simulink model "lab4_S6_7_8_estimation_control"  (R2024b)
settings: Solver=ode23  StartTime=0.0  StopTime=sIn.simulation_time  RelTol=1e-3
values from neighbouring files (symbols this model uses):
  g = 9.81    [balrob_params.m]
  ms22g = 1/g    (= 0.101936799185)    [balrob_params.m]
  Ts = 1e-2    (= 0.01)    [balrob_params.m]
undefined symbols (not defined in the file or in its folder): DiscIntNeverNeededParam, Discrete, drv, feedback, filter, gbox, model, sens, sIn, Time, ua2tau, wheel
libraries: ctrlSharedLib x2
settings Model: Creator=Nihal  LastModifiedBy=Nihal

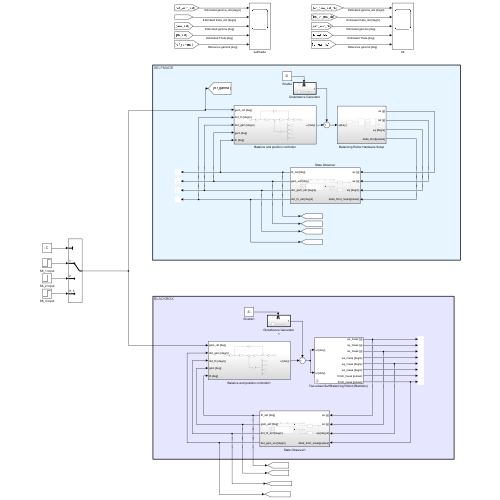
[thumbnail: Simulink's stored preview of the top-level diagram]
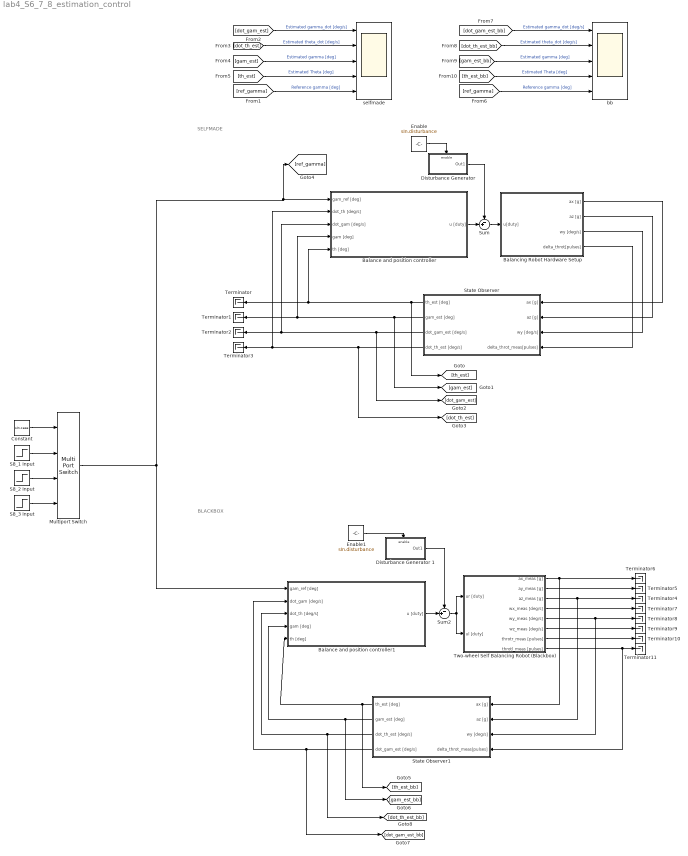
== system lab4_S6_7_8_estimation_control ==
  note: SELFMADE
  note: BLACKBOX
  Balance and position controller : Subsystem
  Balance and position controller1 : Subsystem
  Balancing Robot Hardware Setup : Subsystem
  Constant : Constant  Value=sIn.case
  "Disturbance Generator " : Subsystem  TreatAsAtomicUnit=on
  Disturbance Generator 1 : Subsystem  TreatAsAtomicUnit=on
  Enable : Constant  Value=sIn.disturbance
  Enable1 : Constant  Value=sIn.disturbance
  Multiport Switch : MultiPortSwitch  SaturateOnIntegerOverflow=off  InputSameDT=off
  S8_1 Input : Step  Time=0  After=0  SampleTime=0
  S8_2 Input : Step  Time=0  After=0.1/wheel.r  SampleTime=0
  S8_3 Input : Step  Time=0  After=0.1/wheel.r  SampleTime=0
  State Observer : Subsystem
  State Observer1 : Subsystem
  Sum : Sum  Inputs=-+|
  Sum2 : Sum  Inputs=-+|
  Terminator{,1..11} (12 alike) : Terminator
  "Two-wheel Self Balancing Robot (Blackbox) " : Subsystem  mask(Balancing robot (longitudinal + lateral dynamics)){initState=sIn.bb_ic, Ts=0.01}
      mask prompts: initState "Initial state [gam(0), psi(0), th(0), dot_gam(0), dot_psi(0), dot_th(0)]'"; Ts "Sample time:"
      mask help:
      | Balancing robot dynamic model.
      | Includes both the longitudinal and lateral (yaw) dynamics.
      mask init:
      | %% General parameters and conversion gains
      | 
      | %   gravity acc [m/s^2]
      | g = 9.81;
      | 
      | %   conversion gains
      | rpm2rads = 2*pi/60;         %   [rpm]   -> [rad/s]
      | rads2rpm = 60/2/pi;         %   [rad/s] -> [rpm]
      | rpm2degs = 360/60;          %   [rpm]   -> [deg/s]
      | degs2rpm = 60/360;          %   [deg/s] -> [rpm]
      | deg2rad = pi/180;           %   [deg]   -> [rad]
      | rad2deg = 180/pi;           %   [rad]   -> [deg]
      | g2ms2 = g;                  %   [acc_g] -> [m/s^2]
      | ms22g = 1/g;                %   [m/s^2] -> [acc_g]
      | ozin2Nm = 0.706e-2;         %   [oz*inch] -> [N*m]
      | 
      | 
      | %%  Battery data
      | 
      | %   electrical data
      | batt.UN = 11.1;     %   nominal voltage
      | 
      | 
      | %%  H-bridge PWM voltage driver
      | 
      | drv.Vbus = batt.UN;                     %   H-bridge DC bus voltage  
      | drv.pwm.bits = 8;                       %   PWM resolution [bits]
      | drv.pwm.levels = 2^drv.pwm.bits;        %   PWM levels
      | drv.pwm.Fs = 490;                       %   PWM frequency
      | drv.dutymax = drv.pwm.levels-1;         %   max duty cycle code
      | drv.duty2V = drv.Vbus/drv.dutymax;      %   duty cycle code (0-255) to voltage
      | drv.V2duty = drv.dutymax/drv.Vbus;      %   voltage to duty cycle code (0-255)
      | 
      | 
      | %%  Gearbox data 
      | 
      | gbox.N = 30;            %   reduction ratio
      | 
      | 
      | %%  Sensors data - Hall-effect encoder
      | 
      | %   Hall-effect encoder
      | sens.enc.ppr = 16*4;    %   pulses per rotation at motor side (w/ quadrature decoding)
      | sens.enc.pulse2deg = 360/sens.enc.ppr;
      | sens.enc.pulse2rad = 2*pi/sens.enc.ppr;
      | sens.enc.deg2pulse = sens.enc.ppr/360;
      | sens.enc.rad2pulse = sens.enc.ppr/2/pi;
      | 
      | 
      | %%  Sensors data - MPU6050 (accelerometer + gyro)
      | 
      | %   center of mass (CoM) position
      | sens.mpu.xb = 0;
      | sens.mpu.yb = 0;
      | sens.mpu.zb = 13.5e-3;
      | 
      | %       MPU6050 embedded accelerometer specs
      | sens.mpu.acc.bits = 16;
      | sens.mpu.acc.fs_g = 16;                                                         %   full-scale in "g" units
      | sens.mpu.acc.fs = sens.mpu.acc.fs_g * g2ms2;                                    %   full-scale in [m/s^2] 
      | sens.mpu.acc.g2LSB = floor(2^(sens.mpu.acc.bits-1)/sens.mpu.acc.fs_g);          %   sensitivity [LSB/g]
      | sens.mpu.acc.ms22LSB = sens.mpu.acc.g2LSB * ms22g;                              %   sensitvity [LSB/(m/s^2)]
      | sens.mpu.acc.LSB2g = sens.mpu.acc.fs_g/2^(sens.mpu.acc.bits-1);                 %   output quantization step [g/LSB]
      | sens.mpu.acc.LSB2ms2 = sens.mpu.acc.LSB2g * g2ms2;                              %   output quantization step [ms2/LSB]
      | sens.mpu.acc.bw = 94;                                                           %   output low-pass filter bandwidth
      | sens.mpu.acc.noisestd = 400e-6*sqrt(100);                                       %   output noise std [g-rms]
      | sens.mpu.acc.noisevar = sens.mpu.acc.noisestd^2;                                %   output noise var [g^2]
      | 
      | %       MPU6050 embdedded gyroscope specs
      | sens.mpu.gyro.bits = 16;
      | sens.mpu.gyro.fs_degs = 250;                                                    %   full scale in [deg/s (dps)]
      | sens.mpu.gyro.fs = sens.mpu.gyro.fs_degs * deg2rad;                             %   full scale in [rad/s]
      | sens.mpu.gyro.degs2LSB = floor(2^(sens.mpu.gyro.bits-1)/sens.mpu.gyro.fs_degs);	%   sensitivity [LSB/degs]
      | sens.mpu.gyro.rads2LSB = sens.mpu.gyro.degs2LSB * rad2deg;                      %   sensitivity [LSB/rads] 
      | sens.mpu.gyro.LSB2degs = sens.mpu.gyro.fs_degs/2^(sens.mpu.gyro.bits-1);        %   output quantization step [degs/LSB]
      | sens.mpu.gyro.LSB2rads = sens.mpu.gyro.LSB2degs * deg2rad;                      %   output quantization step [rads/LSB]
      | sens.mpu.gyro.bw = 98;                                                          %   output low-pass filter bandwidth
      | sens.mpu.gyro.noisestd = 5e-3*sqrt(100);                                        %   output noise std [degs-rms]
      | sens.mpu.gyro.noisevar = sens.mpu.acc.noisestd ^2;                              %   output noise var [degs^2]
      mask Help:
      | Riccardo Antonello (antonello@dei.unipd.it)
      | 
      | May 19, 2020
      | 
      | Dept. of Information Engineering, University of Padova
  bb : Scope  NumInputPorts=5
  selfmade : Scope  NumInputPorts=5
  wires:
  Balancing Robot Hardware Setup/4(delta_throt[pulses]) -> State Observer/4(delta_throt_meas[pulses])
  Balancing Robot Hardware Setup/3(wy [deg/s]) -> State Observer/3(wy [deg/s])
  Balancing Robot Hardware Setup/2(az [g]) -> State Observer/2(az [g])
  Balancing Robot Hardware Setup/1(ax [g]) -> State Observer/1(ax [g])
  Multiport Switch/1 -> Balance and position controller1/1(gam_ref [deg]), [ref_gamma], Balance and position controller/1(gam_ref [deg])
  "Two-wheel Self Balancing Robot (Blackbox) "/1(ax_meas [g]) -> State Observer1/1(ax [g]), Terminator6/1
  "Two-wheel Self Balancing Robot (Blackbox) "/2(ay_meas [g]) -> Terminator5/1
  "Two-wheel Self Balancing Robot (Blackbox) "/3(az_meas [g]) -> Terminator4/1, State Observer1/2(az [g])
  "Two-wheel Self Balancing Robot (Blackbox) "/4(wx_meas [deg/s]) -> Terminator7/1
  "Two-wheel Self Balancing Robot (Blackbox) "/5(wy_meas [deg/s]) -> Terminator8/1, State Observer1/3(wy [deg/s])
  "Two-wheel Self Balancing Robot (Blackbox) "/6(wz_meas [deg/s]) -> Terminator9/1
  "Two-wheel Self Balancing Robot (Blackbox) "/7(throtr_meas [pulses]) -> Terminator10/1
  "Two-wheel Self Balancing Robot (Blackbox) "/8(throtl_meas [pulses]) -> State Observer1/4(delta_throt_meas[pulses]), Terminator11/1
  State Observer1/4(dot_gam_est [deg/s]) -> [dot_gam_est_bb], Balance and position controller1/2(dot_gam [deg/s])
  State Observer/2(gam_est [deg]) -> [gam_est], Balance and position controller/4(gam [deg]), Terminator1/1
  State Observer/3(dot_gam_est [deg/s]) -> [dot_gam_est], Terminator2/1, Balance and position controller/3(dot_gam [deg/s])
  State Observer/1(th_est [deg]) -> Balance and position controller/5(th [deg]), Terminator/1, [th_est]
  State Observer/4(dot_th_est [deg/s]) -> [dot_th_est], Terminator3/1, Balance and position controller/2(dot_th [deg/s])
  [ref_gamma] -> selfmade/5  "Reference gamma [deg]"
  [th_est] -> selfmade/4  "Estimated Theta [deg]"
  [gam_est] -> selfmade/3  "Estimated gamma [deg]"
  [dot_th_est] -> selfmade/2  "Estimated theta_dot [deg/s]"
  [dot_gam_est] -> selfmade/1  "Estimated gamma_dot [deg/s]"
  State Observer1/2(gam_est [deg]) -> [gam_est_bb], Balance and position controller1/4(gam [deg])
  State Observer1/1(th_est [deg]) -> [th_est_bb], Balance and position controller1/5(th [deg])
  State Observer1/3(dot_th_est [deg/s]) -> Balance and position controller1/3(dot_th [deg/s]), [dot_th_est_bb]
  [dot_th_est_bb] -> bb/2  "Estimated theta_dot [deg/s]"
  [gam_est_bb] -> bb/3  "Estimated gamma [deg]"
  [ref_gamma] -> bb/5  "Reference gamma [deg]"
  [th_est_bb] -> bb/4  "Estimated Theta [deg]"
  [dot_gam_est_bb] -> bb/1  "Estimated gamma_dot [deg/s]"
  S8_1 Input/1 -> Multiport Switch/2
  S8_2 Input/1 -> Multiport Switch/3
  Constant/1 -> Multiport Switch/1
  Balance and position controller/1(u [duty]) -> Sum/2
  Sum/1 -> Balancing Robot Hardware Setup/1(u[duty])
  "Disturbance Generator "/1(Out1) -> Sum/1
  Enable/1 -> "Disturbance Generator "/Enable
  S8_3 Input/1 -> Multiport Switch/4
  Enable1/1 -> Disturbance Generator 1/Enable
  Balance and position controller1/1(u [duty]) -> Sum2/2
  Sum2/1 -> "Two-wheel Self Balancing Robot (Blackbox) "/2(ul [duty]), "Two-wheel Self Balancing Robot (Blackbox) "/1(ur [duty])
  Disturbance Generator 1/1(Out1) -> Sum2/1

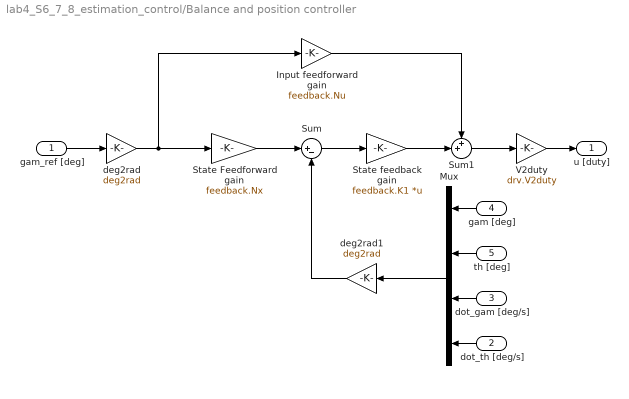
== system lab4_S6_7_8_estimation_control/Balance and position controller ==
  gam_ref [deg] : Inport
  dot_th [deg/s] : Inport  Port=2
  dot_gam [deg/s] : Inport  Port=3
  gam [deg] : Inport  Port=4
  th [deg] : Inport  Port=5
  Input feedforward gain : Gain  Gain=feedback.Nu
  Mux : Mux
  State Feedforward gain : Gain  Gain=feedback.Nx
  State feedback gain : Gain  Gain=feedback.K1  Multiplication=Matrix(K*u)
  Sum : Sum  Inputs=|+-
  Sum1 : Sum  Inputs=++|
  V2duty : Gain  Gain=drv.V2duty
  deg2rad : Gain  Gain=deg2rad
  deg2rad1 : Gain  Gain=deg2rad
  u [duty] : Outport
  wires:
  gam_ref [deg]/1 -> deg2rad/1
  deg2rad/1 -> Input feedforward gain/1, State Feedforward gain/1
  State Feedforward gain/1 -> Sum/1
  deg2rad1/1 -> Sum/2
  Mux/1 -> deg2rad1/1
  gam [deg]/1 -> Mux/1
  dot_th [deg/s]/1 -> Mux/4
  dot_gam [deg/s]/1 -> Mux/3
  th [deg]/1 -> Mux/2
  Sum/1 -> State feedback gain/1
  State feedback gain/1 -> Sum1/2
  Input feedforward gain/1 -> Sum1/1
  Sum1/1 -> V2duty/1
  V2duty/1 -> u [duty]/1

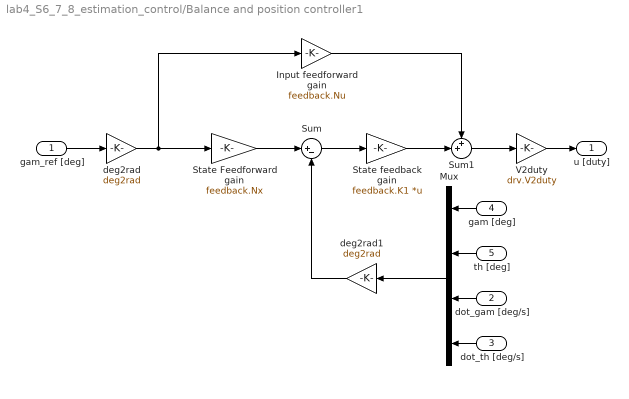
== system lab4_S6_7_8_estimation_control/Balance and position controller1 ==
  gam_ref [deg] : Inport
  dot_gam [deg/s] : Inport  Port=2
  dot_th [deg/s] : Inport  Port=3
  gam [deg] : Inport  Port=4
  th [deg] : Inport  Port=5
  Input feedforward gain : Gain  Gain=feedback.Nu
  Mux : Mux
  State Feedforward gain : Gain  Gain=feedback.Nx
  State feedback gain : Gain  Gain=feedback.K1  Multiplication=Matrix(K*u)
  Sum : Sum  Inputs=|+-
  Sum1 : Sum  Inputs=++|
  V2duty : Gain  Gain=drv.V2duty
  deg2rad : Gain  Gain=deg2rad
  deg2rad1 : Gain  Gain=deg2rad
  u [duty] : Outport
  wires:
  gam_ref [deg]/1 -> deg2rad/1
  deg2rad/1 -> Input feedforward gain/1, State Feedforward gain/1
  State Feedforward gain/1 -> Sum/1
  deg2rad1/1 -> Sum/2
  Mux/1 -> deg2rad1/1
  gam [deg]/1 -> Mux/1
  dot_th [deg/s]/1 -> Mux/4
  dot_gam [deg/s]/1 -> Mux/3
  th [deg]/1 -> Mux/2
  Sum/1 -> State feedback gain/1
  State feedback gain/1 -> Sum1/2
  Input feedforward gain/1 -> Sum1/1
  Sum1/1 -> V2duty/1
  V2duty/1 -> u [duty]/1

== system lab4_S6_7_8_estimation_control/Balancing Robot Hardware Setup ==
  u[duty] : Inport
  Electromechanical Dynamics : Subsystem
  Encoder : Subsystem
  Motion Processing Unit (MPU) : Subsystem
  Voltage driver : Subsystem
  ax [g] : Outport
  az [g] : Outport  Port=2
  wy [deg/s] : Outport  Port=3
  delta_throt[pulses] : Outport  Port=4
  wires:
  Voltage driver/1(u[V]) -> Electromechanical Dynamics/1(ua [V])
  Electromechanical Dynamics/1(q [deg]) -> Encoder/1(q[deg]), Motion Processing Unit (MPU)/1(q [deg])
  u[duty]/1 -> Voltage driver/1(u[duty])
  Electromechanical Dynamics/3(ddot_q [deg/s^2]) -> Motion Processing Unit (MPU)/3(ddot_q [deg/s^2])
  Motion Processing Unit (MPU)/3(wy [deg/s]) -> wy [deg/s]/1
  Electromechanical Dynamics/2(dot_q [deg/s]) -> Motion Processing Unit (MPU)/2(dot_q [deg/s])
  Motion Processing Unit (MPU)/2(az [g]) -> az [g]/1
  Motion Processing Unit (MPU)/1(ax [g]) -> ax [g]/1
  Encoder/1(delta_throt[pulses]) -> delta_throt[pulses]/1

== system lab4_S6_7_8_estimation_control/Disturbance Generator  ==
  Enable : EnablePort
  Step : Step  Time=10  After=5/drv.duty2V  SampleTime=0
  Out1 : Outport
  wires:
  Step/1 -> Out1/1

== system lab4_S6_7_8_estimation_control/Disturbance Generator 1 ==
  Enable : EnablePort
  Step : Step  Time=10  After=5/drv.duty2V  SampleTime=0
  Out1 : Outport
  wires:
  Step/1 -> Out1/1

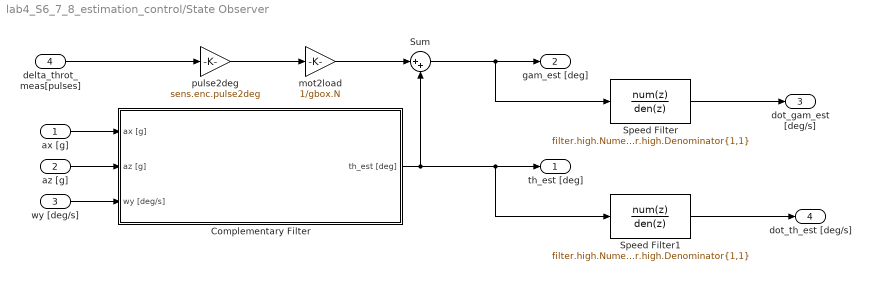
== system lab4_S6_7_8_estimation_control/State Observer ==
  ax [g] : Inport
  az [g] : Inport  Port=2
  wy [deg/s] : Inport  Port=3
  delta_throt_meas[pulses] : Inport  Port=4
  Complementary Filter : Subsystem
  Speed Filter : DiscreteFilter  Numerator=filter.high.Numerator{1,1}  Denominator=filter.high.Denominator{1,1}
  Speed Filter1 : DiscreteFilter  Numerator=filter.high.Numerator{1,1}  Denominator=filter.high.Denominator{1,1}
  Sum : Sum  Inputs=|++
  mot2load : Gain  Gain=1/gbox.N
  pulse2deg : Gain  Gain=sens.enc.pulse2deg
  th_est [deg] : Outport
  gam_est [deg] : Outport  Port=2
  dot_gam_est [deg/s] : Outport  Port=3
  dot_th_est [deg/s] : Outport  Port=4
  wires:
  wy [deg/s]/1 -> Complementary Filter/3(wy [deg/s])
  az [g]/1 -> Complementary Filter/2(az [g])
  ax [g]/1 -> Complementary Filter/1(ax [g])
  Complementary Filter/1(th_est [deg]) -> Sum/2, Speed Filter1/1, th_est [deg]/1
  delta_throt_meas[pulses]/1 -> pulse2deg/1
  pulse2deg/1 -> mot2load/1
  mot2load/1 -> Sum/1
  Sum/1 -> Speed Filter/1, gam_est [deg]/1
  Speed Filter1/1 -> dot_th_est [deg/s]/1
  Speed Filter/1 -> dot_gam_est [deg/s]/1

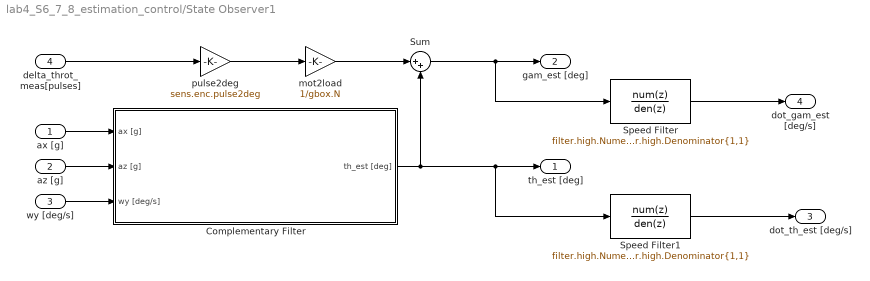
== system lab4_S6_7_8_estimation_control/State Observer1 ==
  ax [g] : Inport
  az [g] : Inport  Port=2
  wy [deg/s] : Inport  Port=3
  delta_throt_meas[pulses] : Inport  Port=4
  Complementary Filter : Subsystem
  Speed Filter : DiscreteFilter  Numerator=filter.high.Numerator{1,1}  Denominator=filter.high.Denominator{1,1}
  Speed Filter1 : DiscreteFilter  Numerator=filter.high.Numerator{1,1}  Denominator=filter.high.Denominator{1,1}
  Sum : Sum  Inputs=|++
  mot2load : Gain  Gain=1/gbox.N
  pulse2deg : Gain  Gain=sens.enc.pulse2deg
  th_est [deg] : Outport
  gam_est [deg] : Outport  Port=2
  dot_th_est [deg/s] : Outport  Port=3
  dot_gam_est [deg/s] : Outport  Port=4
  wires:
  wy [deg/s]/1 -> Complementary Filter/3(wy [deg/s])
  az [g]/1 -> Complementary Filter/2(az [g])
  ax [g]/1 -> Complementary Filter/1(ax [g])
  Complementary Filter/1(th_est [deg]) -> Sum/2, Speed Filter1/1, th_est [deg]/1
  delta_throt_meas[pulses]/1 -> pulse2deg/1
  pulse2deg/1 -> mot2load/1
  mot2load/1 -> Sum/1
  Sum/1 -> Speed Filter/1, gam_est [deg]/1
  Speed Filter1/1 -> dot_th_est [deg/s]/1
  Speed Filter/1 -> dot_gam_est [deg/s]/1

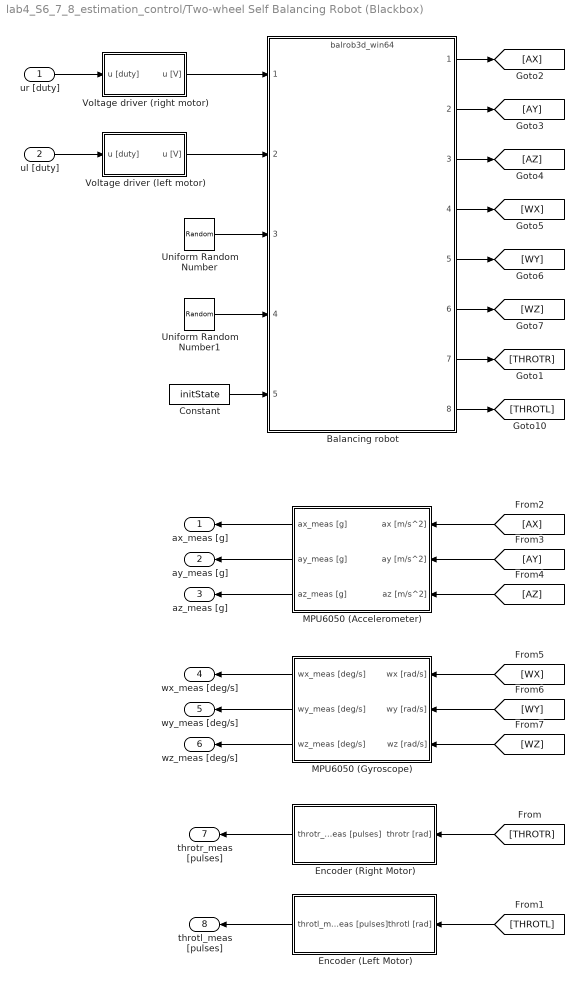
== system lab4_S6_7_8_estimation_control/Two-wheel Self Balancing Robot (Blackbox)  ==
  ur [duty] : Inport
  ul [duty] : Inport  Port=2
  Balancing robot : ModelReference  ModelNameDialog=balrob3d_win64.slxp  ModelReferenceVersion=1.741  CopyOfModelProtected=on
  Constant : Constant  Value=initState
  Encoder (Left Motor) : Subsystem
  Encoder (Right Motor) : Subsystem
  MPU6050 (Accelerometer) : Subsystem
  MPU6050 (Gyroscope) : Subsystem
  Uniform Random Number : UniformRandomNumber  Minimum=0.7  Maximum=1.3  SampleTime=1
  Uniform Random Number1 : UniformRandomNumber  Minimum=0.7  Maximum=1.3  Seed=10  SampleTime=1
  Voltage driver (left motor) : Subsystem
  Voltage driver (right motor) : Subsystem
  ax_meas [g] : Outport
  ay_meas [g] : Outport  Port=2
  az_meas [g] : Outport  Port=3
  wx_meas [deg/s] : Outport  Port=4
  wy_meas [deg/s] : Outport  Port=5
  wz_meas [deg/s] : Outport  Port=6
  throtr_meas [pulses] : Outport  Port=7
  throtl_meas [pulses] : Outport  Port=8
  wires:
  ur [duty]/1 -> Voltage driver (right motor)/1(u [duty])
  [WX] -> MPU6050 (Gyroscope)/1(wx [rad/s])
  Balancing robot/2 -> [AY]
  Balancing robot/4 -> [WX]
  Balancing robot/8 -> [THROTL]
  Balancing robot/1 -> [AX]
  [THROTL] -> Encoder (Left Motor)/1(throtl [rad])
  Balancing robot/6 -> [WZ]
  Balancing robot/7 -> [THROTR]
  Balancing robot/5 -> [WY]
  [AX] -> MPU6050 (Accelerometer)/1(ax [m/s^2])
  [WY] -> MPU6050 (Gyroscope)/2(wy [rad/s])
  Balancing robot/3 -> [AZ]
  [WZ] -> MPU6050 (Gyroscope)/3(wz [rad/s])
  [AZ] -> MPU6050 (Accelerometer)/3(az [m/s^2])
  [THROTR] -> Encoder (Right Motor)/1(throtr [rad])
  ul [duty]/1 -> Voltage driver (left motor)/1(u [duty])
  [AY] -> MPU6050 (Accelerometer)/2(ay [m/s^2])
  MPU6050 (Accelerometer)/1(ax_meas [g]) -> ax_meas [g]/1
  MPU6050 (Accelerometer)/2(ay_meas [g]) -> ay_meas [g]/1
  MPU6050 (Accelerometer)/3(az_meas [g]) -> az_meas [g]/1
  MPU6050 (Gyroscope)/1(wx_meas [deg/s]) -> wx_meas [deg/s]/1
  MPU6050 (Gyroscope)/2(wy_meas [deg/s]) -> wy_meas [deg/s]/1
  MPU6050 (Gyroscope)/3(wz_meas [deg/s]) -> wz_meas [deg/s]/1
  Encoder (Right Motor)/1(throtr_meas [pulses]) -> throtr_meas [pulses]/1
  Encoder (Left Motor)/1(throtl_meas [pulses]) -> throtl_meas [pulses]/1
  Voltage driver (right motor)/1(u [V]) -> Balancing robot/1
  Voltage driver (left motor)/1(u [V]) -> Balancing robot/2
  Uniform Random Number/1 -> Balancing robot/3
  Uniform Random Number1/1 -> Balancing robot/4
  Constant/1 -> Balancing robot/5

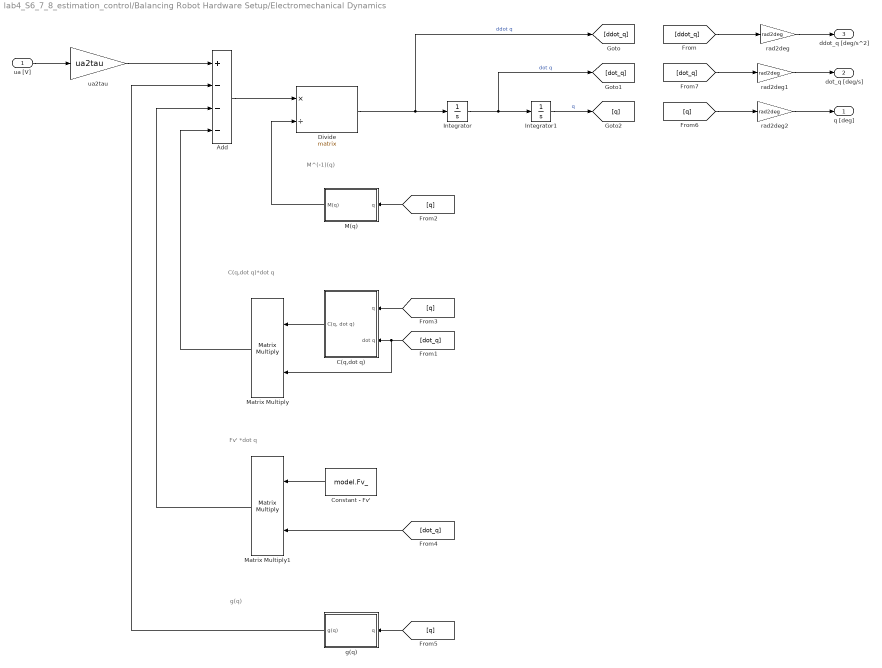
== system lab4_S6_7_8_estimation_control/Balancing Robot Hardware Setup/Electromechanical Dynamics ==
  note: g(q)
  note: Fv' *dot q
  note: C(q,dot q)*dot q
  note: M^(-1)(q)
  ua [V] : Inport
  Add : Sum  Inputs=+---
  C(q,dot q) : Subsystem
  Constant - Fv' : Constant  Value=model.Fv_
  Divide : Product  Inputs=*/  Multiplication=Matrix(*)
  Integrator : Integrator  InitialCondition=sIn.x0(3:4)
  Integrator1 : Integrator  InitialCondition=sIn.x0(1:2)
  M(q) : Subsystem
  Matrix Multiply : Product  Multiplication=Matrix(*)
  Matrix Multiply1 : Product  Multiplication=Matrix(*)
  g(q) : Subsystem
  rad2deg : Gain  Gain=rad2deg
  rad2deg1 : Gain  Gain=rad2deg
  rad2deg2 : Gain  Gain=rad2deg
  ua2tau : Gain  Gain=ua2tau
  q [deg] : Outport
  dot_q [deg/s] : Outport  Port=2
  ddot_q [deg/s^2] : Outport  Port=3
  wires:
  ua [V]/1 -> ua2tau/1
  ua2tau/1 -> Add/1
  Add/1 -> Divide/1
  Divide/1 -> [ddot_q], Integrator/1  "ddot q"
  Integrator/1 -> [dot_q], Integrator1/1  "dot q"
  Integrator1/1 -> [q]  "q"
  [q] -> M(q)/1(q)
  M(q)/1(M(q)) -> Divide/2
  C(q,dot q)/1("C(q, dot q)") -> Matrix Multiply/1
  [dot_q] -> Matrix Multiply/2, C(q,dot q)/2(dot q)
  [q] -> C(q,dot q)/1(q)
  Constant - Fv'/1 -> Matrix Multiply1/1
  [dot_q] -> Matrix Multiply1/2
  [q] -> g(q)/1(q)
  Matrix Multiply/1 -> Add/4
  Matrix Multiply1/1 -> Add/3
  g(q)/1(g(q)) -> Add/2
  [ddot_q] -> rad2deg/1
  [dot_q] -> rad2deg1/1
  [q] -> rad2deg2/1
  rad2deg2/1 -> q [deg]/1
  rad2deg/1 -> ddot_q [deg/s^2]/1
  rad2deg1/1 -> dot_q [deg/s]/1

== system lab4_S6_7_8_estimation_control/Balancing Robot Hardware Setup/Encoder ==
  q[deg] : Inport
  Add : Sum  Inputs=+-
  Demux : Demux  Outputs=2
  Quantizer : Quantizer  QuantizationInterval=sens.enc.pulse2deg
  Zero-Order Hold : ZeroOrderHold  SampleTime=Ts
  deg2pulse : Gain  Gain=sens.enc.deg2pulse
  load2mot : Gain  Gain=gbox.N
  delta_throt[pulses] : Outport
  wires:
  Add/1 -> load2mot/1
  Zero-Order Hold/1 -> Quantizer/1
  q[deg]/1 -> Demux/1
  Demux/2 -> Add/2  "th"
  Quantizer/1 -> deg2pulse/1
  Demux/1 -> Add/1  "gam"
  deg2pulse/1 -> delta_throt[pulses]/1
  load2mot/1 -> Zero-Order Hold/1  "delta_throt"

== system lab4_S6_7_8_estimation_control/Balancing Robot Hardware Setup/Motion Processing Unit (MPU) ==
  q [deg] : Inport
  dot_q [deg/s] : Inport  Port=2
  ddot_q [deg/s^2] : Inport  Port=3
  Accelerometer : Subsystem
  Gyroscope : Subsystem
  ax [g] : Outport
  az [g] : Outport  Port=2
  wy [deg/s] : Outport  Port=3
  wires:
  Gyroscope/1(wy [deg/s]) -> wy [deg/s]/1
  ddot_q [deg/s^2]/1 -> Accelerometer/3(ddot_q [deg/s^2])
  q [deg]/1 -> Accelerometer/1(q [deg])
  Accelerometer/1(ax [g]) -> ax [g]/1
  dot_q [deg/s]/1 -> Gyroscope/1(dot_q [deg/s]), Accelerometer/2(dot_q [deg/s])
  Accelerometer/2(az [g]) -> az [g]/1

== system lab4_S6_7_8_estimation_control/Balancing Robot Hardware Setup/Voltage driver ==
  u[duty] : Inport
  Duty Saturation : Saturate  UpperLimit=drv.dutymax  LowerLimit=-drv.dutymax
  Rounding function : Rounding  Operator=fix
  Voltage saturation : Saturate  UpperLimit=drv.Vbus  LowerLimit=-drv.Vbus
  Zero-Order Hold : ZeroOrderHold  SampleTime=Ts
  duty2V : Gain  Gain=drv.duty2V
  u[V] : Outport
  wires:
  Voltage saturation/1 -> Zero-Order Hold/1
  duty2V/1 -> Voltage saturation/1
  Rounding function/1 -> duty2V/1
  Zero-Order Hold/1 -> u[V]/1
  Duty Saturation/1 -> Rounding function/1
  u[duty]/1 -> Duty Saturation/1

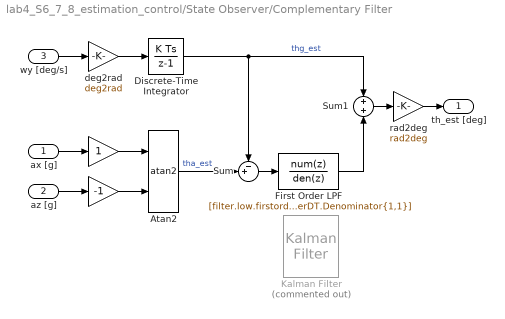
== system lab4_S6_7_8_estimation_control/State Observer/Complementary Filter ==
  ax [g] : Inport
  az [g] : Inport  Port=2
  wy [deg/s] : Inport  Port=3
  " " : Gain
  "   " : Gain  Gain=-1
  Atan2 : Trigonometry  Operator=atan2
  Discrete-Time Integrator : DiscreteIntegrator  InitialCondition=sIn.x0(2)  SampleTime=sIn.Ts  ICPrevOutput=DiscIntNeverNeededParam  ICPrevScaledInput=DiscIntNeverNeededParam
  First Order LPF : DiscreteTransferFcn  Numerator=[filter.low.firstorderDT.Numerator{1,1}]  Denominator=[filter.low.firstorderDT.Denominator{1,1}]
  Kalman Filter : ctrlSharedLib/Kalman Filter  Commented=on  TimeDomain=Discrete-Time  UseCurrentEstimator=on  ModelSource=LTI State-Space Variable  ModelSourceVariable=ss(0.95,1,1,0,1)  A=0.95  B=1  C=1  D=0  NumberOfStates=1  NumberOfInputs=1  NumberOfOutputs=1  InitialEstimateSource=Dialog  X0=0  P0=10  UseK=off  UseGH=off  NumberOfProcessNoiseInputs=1  G=1  TimeInvariantG=on  H=0  TimeInvariantH=on  Q=0.05  TimeInvariantQ=on  R=1  TimeInvariantR=on  N=0  TimeInvariantN=on  AddInputPort=on  AddEnablePort=off  OutputEstimatedY=off  OutputP=off  Ts=-1
  Sum : Sum  Inputs=-+|
  Sum1 : Sum  Inputs=+|+
  deg2rad : Gain  Gain=deg2rad
  rad2deg : Gain  Gain=rad2deg
  th_est [deg] : Outport
  wires:
  wy [deg/s]/1 -> deg2rad/1
  deg2rad/1 -> Discrete-Time Integrator/1
  az [g]/1 -> "   "/1
  ax [g]/1 -> " "/1
  "   "/1 -> Atan2/2
  " "/1 -> Atan2/1
  Atan2/1 -> Sum/2  "tha_est"
  Discrete-Time Integrator/1 -> Sum1/1, Sum/1  "thg_est"
  Sum/1 -> First Order LPF/1
  First Order LPF/1 -> Sum1/2
  Sum1/1 -> rad2deg/1
  rad2deg/1 -> th_est [deg]/1

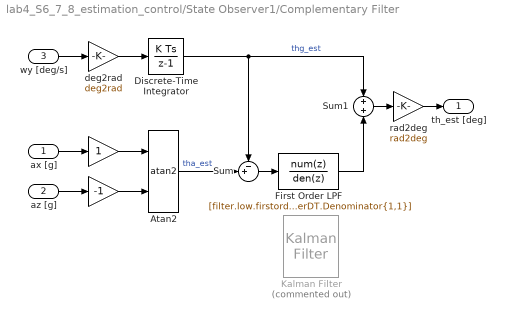
== system lab4_S6_7_8_estimation_control/State Observer1/Complementary Filter ==
  ax [g] : Inport
  az [g] : Inport  Port=2
  wy [deg/s] : Inport  Port=3
  " " : Gain
  "   " : Gain  Gain=-1
  Atan2 : Trigonometry  Operator=atan2
  Discrete-Time Integrator : DiscreteIntegrator  InitialCondition=sIn.x0(2)  SampleTime=sIn.Ts  ICPrevOutput=DiscIntNeverNeededParam  ICPrevScaledInput=DiscIntNeverNeededParam
  First Order LPF : DiscreteTransferFcn  Numerator=[filter.low.firstorderDT.Numerator{1,1}]  Denominator=[filter.low.firstorderDT.Denominator{1,1}]
  Kalman Filter : ctrlSharedLib/Kalman Filter  Commented=on  TimeDomain=Discrete-Time  UseCurrentEstimator=on  ModelSource=LTI State-Space Variable  ModelSourceVariable=ss(0.95,1,1,0,1)  A=0.95  B=1  C=1  D=0  NumberOfStates=1  NumberOfInputs=1  NumberOfOutputs=1  InitialEstimateSource=Dialog  X0=0  P0=10  UseK=off  UseGH=off  NumberOfProcessNoiseInputs=1  G=1  TimeInvariantG=on  H=0  TimeInvariantH=on  Q=0.05  TimeInvariantQ=on  R=1  TimeInvariantR=on  N=0  TimeInvariantN=on  AddInputPort=on  AddEnablePort=off  OutputEstimatedY=off  OutputP=off  Ts=-1
  Sum : Sum  Inputs=-+|
  Sum1 : Sum  Inputs=+|+
  deg2rad : Gain  Gain=deg2rad
  rad2deg : Gain  Gain=rad2deg
  th_est [deg] : Outport
  wires:
  wy [deg/s]/1 -> deg2rad/1
  deg2rad/1 -> Discrete-Time Integrator/1
  az [g]/1 -> "   "/1
  ax [g]/1 -> " "/1
  "   "/1 -> Atan2/2
  " "/1 -> Atan2/1
  Atan2/1 -> Sum/2  "tha_est"
  Discrete-Time Integrator/1 -> Sum1/1, Sum/1  "thg_est"
  Sum/1 -> First Order LPF/1
  First Order LPF/1 -> Sum1/2
  Sum1/1 -> rad2deg/1
  rad2deg/1 -> th_est [deg]/1

== system lab4_S6_7_8_estimation_control/Two-wheel Self Balancing Robot (Blackbox) /Encoder (Left Motor) ==
  throtl [rad] : Inport
  Quantizer : Quantizer  QuantizationInterval=sens.enc.pulse2rad
  Zero-Order Hold : ZeroOrderHold  SampleTime=Ts
  rad2pulse : Gain  Gain=sens.enc.rad2pulse
  throtl_meas [pulses] : Outport
  wires:
  Quantizer/1 -> rad2pulse/1
  Zero-Order Hold/1 -> Quantizer/1
  throtl [rad]/1 -> Zero-Order Hold/1
  rad2pulse/1 -> throtl_meas [pulses]/1

== system lab4_S6_7_8_estimation_control/Two-wheel Self Balancing Robot (Blackbox) /Encoder (Right Motor) ==
  throtr [rad] : Inport
  Quantizer : Quantizer  QuantizationInterval=sens.enc.pulse2rad
  Zero-Order Hold : ZeroOrderHold  SampleTime=Ts
  rad2pulse : Gain  Gain=sens.enc.rad2pulse
  throtr_meas [pulses] : Outport
  wires:
  throtr [rad]/1 -> Zero-Order Hold/1
  Zero-Order Hold/1 -> Quantizer/1
  Quantizer/1 -> rad2pulse/1
  rad2pulse/1 -> throtr_meas [pulses]/1

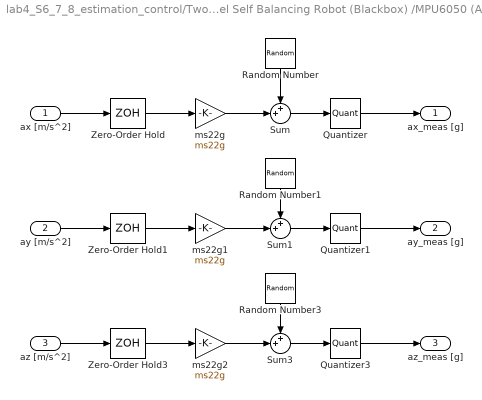
== system lab4_S6_7_8_estimation_control/Two-wheel Self Balancing Robot (Blackbox) /MPU6050 (Accelerometer) ==
  ax [m/s^2] : Inport
  ay [m/s^2] : Inport  Port=2
  az [m/s^2] : Inport  Port=3
  Quantizer : Quantizer  QuantizationInterval=sens.mpu.acc.LSB2g
  Quantizer1 : Quantizer  QuantizationInterval=sens.mpu.acc.LSB2g
  Quantizer3 : Quantizer  QuantizationInterval=sens.mpu.acc.LSB2g
  Random Number : RandomNumber  Variance=sens.mpu.acc.noisevar  Seed=1  SampleTime=Ts
  Random Number1 : RandomNumber  Variance=sens.mpu.acc.noisevar  Seed=10  SampleTime=Ts
  Random Number3 : RandomNumber  Variance=sens.mpu.acc.noisevar  Seed=100  SampleTime=Ts
  Sum : Sum  Inputs=++|
  Sum1 : Sum  Inputs=++|
  Sum3 : Sum  Inputs=++|
  Zero-Order Hold : ZeroOrderHold  SampleTime=Ts
  Zero-Order Hold1 : ZeroOrderHold  SampleTime=Ts
  Zero-Order Hold3 : ZeroOrderHold  SampleTime=Ts
  ms22g : Gain  Gain=ms22g
  ms22g1 : Gain  Gain=ms22g
  ms22g2 : Gain  Gain=ms22g
  ax_meas [g] : Outport
  ay_meas [g] : Outport  Port=2
  az_meas [g] : Outport  Port=3
  wires:
  ax [m/s^2]/1 -> Zero-Order Hold/1
  Zero-Order Hold1/1 -> ms22g1/1
  Sum1/1 -> Quantizer1/1
  ms22g/1 -> Sum/2
  ay [m/s^2]/1 -> Zero-Order Hold1/1
  Sum3/1 -> Quantizer3/1
  ms22g1/1 -> Sum1/2
  Random Number1/1 -> Sum1/1
  Random Number/1 -> Sum/1
  Sum/1 -> Quantizer/1
  Random Number3/1 -> Sum3/1
  ms22g2/1 -> Sum3/2
  Zero-Order Hold3/1 -> ms22g2/1
  az [m/s^2]/1 -> Zero-Order Hold3/1
  Zero-Order Hold/1 -> ms22g/1
  Quantizer/1 -> ax_meas [g]/1
  Quantizer1/1 -> ay_meas [g]/1
  Quantizer3/1 -> az_meas [g]/1

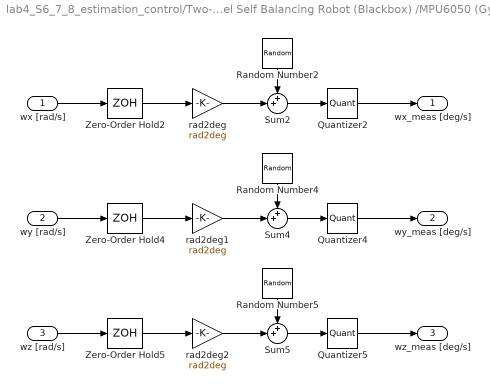
== system lab4_S6_7_8_estimation_control/Two-wheel Self Balancing Robot (Blackbox) /MPU6050 (Gyroscope) ==
  wx [rad/s] : Inport
  wy [rad/s] : Inport  Port=2
  wz [rad/s] : Inport  Port=3
  Quantizer2 : Quantizer  QuantizationInterval=sens.mpu.gyro.LSB2degs
  Quantizer4 : Quantizer  QuantizationInterval=sens.mpu.gyro.LSB2degs
  Quantizer5 : Quantizer  QuantizationInterval=sens.mpu.gyro.LSB2degs
  Random Number2 : RandomNumber  Variance=sens.mpu.gyro.noisevar  Seed=2  SampleTime=Ts
  Random Number4 : RandomNumber  Variance=sens.mpu.gyro.noisevar  Seed=20  SampleTime=Ts
  Random Number5 : RandomNumber  Variance=sens.mpu.gyro.noisevar  Seed=200  SampleTime=Ts
  Sum2 : Sum  Inputs=++|
  Sum4 : Sum  Inputs=++|
  Sum5 : Sum  Inputs=++|
  Zero-Order Hold2 : ZeroOrderHold  SampleTime=Ts
  Zero-Order Hold4 : ZeroOrderHold  SampleTime=Ts
  Zero-Order Hold5 : ZeroOrderHold  SampleTime=Ts
  rad2deg : Gain  Gain=rad2deg
  rad2deg1 : Gain  Gain=rad2deg
  rad2deg2 : Gain  Gain=rad2deg
  wx_meas [deg/s] : Outport
  wy_meas [deg/s] : Outport  Port=2
  wz_meas [deg/s] : Outport  Port=3
  wires:
  Random Number2/1 -> Sum2/1
  Sum2/1 -> Quantizer2/1
  Quantizer2/1 -> wx_meas [deg/s]/1
  Zero-Order Hold5/1 -> rad2deg2/1
  Sum4/1 -> Quantizer4/1
  rad2deg/1 -> Sum2/2
  rad2deg2/1 -> Sum5/2
  Random Number5/1 -> Sum5/1
  Zero-Order Hold4/1 -> rad2deg1/1
  Sum5/1 -> Quantizer5/1
  Random Number4/1 -> Sum4/1
  Zero-Order Hold2/1 -> rad2deg/1
  Quantizer5/1 -> wz_meas [deg/s]/1
  wz [rad/s]/1 -> Zero-Order Hold5/1
  wx [rad/s]/1 -> Zero-Order Hold2/1
  rad2deg1/1 -> Sum4/2
  Quantizer4/1 -> wy_meas [deg/s]/1
  wy [rad/s]/1 -> Zero-Order Hold4/1

== system lab4_S6_7_8_estimation_control/Two-wheel Self Balancing Robot (Blackbox) /Voltage driver (left motor) ==
  u [duty] : Inport
  Rounding Function : Rounding  Operator=fix
  Unit Delay : UnitDelay  SampleTime=1/drv.pwm.Fs  HasFrameUpgradeWarning=on
  Zero-Order Hold : ZeroOrderHold  SampleTime=Ts
  duty saturation : Saturate  UpperLimit=255  LowerLimit=-255
  duty2V : Gain  Gain=drv.duty2V
  voltage saturation : Saturate  UpperLimit=drv.Vbus  LowerLimit=-drv.Vbus
  u [V] : Outport
  wires:
  Zero-Order Hold/1 -> Unit Delay/1
  u [duty]/1 -> duty saturation/1
  voltage saturation/1 -> Zero-Order Hold/1
  duty saturation/1 -> Rounding Function/1
  Rounding Function/1 -> duty2V/1
  duty2V/1 -> voltage saturation/1
  Unit Delay/1 -> u [V]/1

== system lab4_S6_7_8_estimation_control/Two-wheel Self Balancing Robot (Blackbox) /Voltage driver (right motor) ==
  u [duty] : Inport
  Rounding Function : Rounding  Operator=fix
  Unit Delay : UnitDelay  SampleTime=1/drv.pwm.Fs  HasFrameUpgradeWarning=on
  Zero-Order Hold : ZeroOrderHold  SampleTime=Ts
  duty saturation : Saturate  UpperLimit=255  LowerLimit=-255
  duty2V : Gain  Gain=drv.duty2V
  voltage saturation : Saturate  UpperLimit=drv.Vbus  LowerLimit=-drv.Vbus
  u [V] : Outport
  wires:
  u [duty]/1 -> duty saturation/1
  duty saturation/1 -> Rounding Function/1
  Zero-Order Hold/1 -> Unit Delay/1
  voltage saturation/1 -> Zero-Order Hold/1
  Rounding Function/1 -> duty2V/1
  duty2V/1 -> voltage saturation/1
  Unit Delay/1 -> u [V]/1

== system lab4_S6_7_8_estimation_control/Balancing Robot Hardware Setup/Electromechanical Dynamics/C(q,dot q) ==
  q : Inport
  dot q : Inport  Port=2
  C12(q dotq) : Fcn  Expr=model.C12_fact*sin(u(1))*u(2)
  Constant : Constant  Value=0
  Matrix Concatenate : Concatenate  Mode=Multidimensional array  ConcatenateDimension=2
  Mux : Mux  Inputs=2
  Mux1 : Mux  Inputs=2
  Mux2 : Mux  Inputs=2
  Selector : Selector  InputPortWidth=2  IndexOptions=Index vector (dialog)  Indices=2  OutputSizes=1
  Selector1 : Selector  InputPortWidth=2  IndexOptions=Index vector (dialog)  Indices=2  OutputSizes=1
  "C(q, dot q)" : Outport
  wires:
  Matrix Concatenate/1 -> "C(q, dot q)"/1
  Mux/1 -> Matrix Concatenate/2
  Mux1/1 -> Matrix Concatenate/1
  Selector/1 -> Mux2/1
  q/1 -> Selector/1
  dot q/1 -> Selector1/1
  Constant/1 -> Mux/2, Mux1/2, Mux1/1
  Selector1/1 -> Mux2/2
  Mux2/1 -> C12(q dotq)/1
  C12(q dotq)/1 -> Mux/1

== system lab4_S6_7_8_estimation_control/Balancing Robot Hardware Setup/Electromechanical Dynamics/M(q) ==
  q : Inport
  Constant - M1 : Constant  Value=model.M22
  Constant - M11 : Constant  Value=model.M11
  Fcn : Fcn  Expr=model.M12_add + model.M12_fact*cos(u)
  Matrix Concatenate : Concatenate  Mode=Multidimensional array  ConcatenateDimension=2
  Mux : Mux  Inputs=2
  Mux1 : Mux  Inputs=2
  Selector : Selector  InputPortWidth=2  IndexOptions=Index vector (dialog)  Indices=2  OutputSizes=1
  M(q) : Outport
  wires:
  q/1 -> Selector/1
  Selector/1 -> Fcn/1
  Constant - M1/1 -> Mux/2
  Constant - M11/1 -> Mux1/1
  Fcn/1 -> Mux/1, Mux1/2
  Mux1/1 -> Matrix Concatenate/1
  Mux/1 -> Matrix Concatenate/2
  Matrix Concatenate/1 -> M(q)/1

== system lab4_S6_7_8_estimation_control/Balancing Robot Hardware Setup/Electromechanical Dynamics/g(q) ==
  q : Inport
  Constant : Constant  Value=0
  Mux1 : Mux  Inputs=2
  Selector : Selector  InputPortWidth=2  IndexOptions=Index vector (dialog)  Indices=2  OutputSizes=1
  g2(q) : Fcn  Expr=model.g2_fact*sin(u)
  g(q) : Outport
  wires:
  Selector/1 -> g2(q)/1
  Constant/1 -> Mux1/1
  q/1 -> Selector/1
  g2(q)/1 -> Mux1/2
  Mux1/1 -> g(q)/1

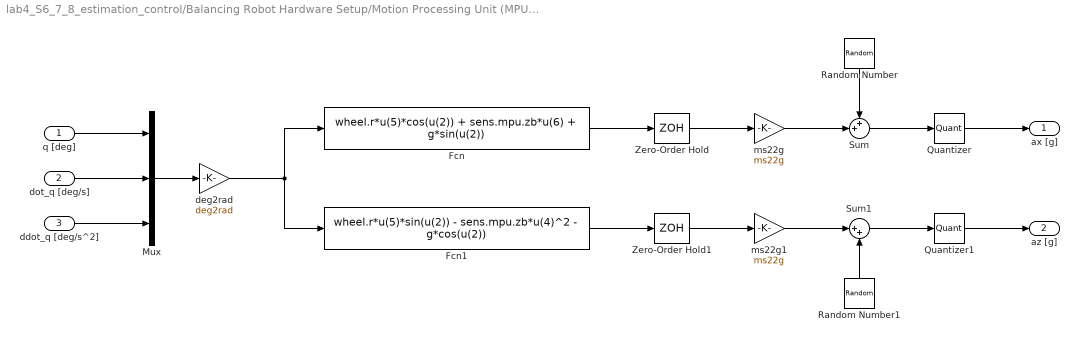
== system lab4_S6_7_8_estimation_control/Balancing Robot Hardware Setup/Motion Processing Unit (MPU)/Accelerometer ==
  q [deg] : Inport
  dot_q [deg/s] : Inport  Port=2
  ddot_q [deg/s^2] : Inport  Port=3
  Fcn : Fcn  Expr=wheel.r*u(5)*cos(u(2)) + sens.mpu.zb*u(6) + g*sin(u(2))
  Fcn1 : Fcn  Expr=wheel.r*u(5)*sin(u(2)) - sens.mpu.zb*u(4)^2 - g*cos(u(2))
  Mux : Mux  Inputs=3
  Quantizer : Quantizer  QuantizationInterval=sens.mpu.acc.LSB2g
  Quantizer1 : Quantizer  QuantizationInterval=sens.mpu.acc.LSB2g
  Random Number : RandomNumber  Variance=sens.mpu.acc.noisevar  SampleTime=Ts
  Random Number1 : RandomNumber  Variance=sens.mpu.acc.noisevar  SampleTime=Ts
  Sum : Sum  Inputs=++|
  Sum1 : Sum  Inputs=|++
  Zero-Order Hold : ZeroOrderHold  SampleTime=Ts
  Zero-Order Hold1 : ZeroOrderHold  SampleTime=Ts
  deg2rad : Gain  Gain=deg2rad
  ms22g : Gain  Gain=ms22g
  ms22g1 : Gain  Gain=ms22g
  ax [g] : Outport
  az [g] : Outport  Port=2
  wires:
  q [deg]/1 -> Mux/1
  dot_q [deg/s]/1 -> Mux/2
  ddot_q [deg/s^2]/1 -> Mux/3
  Mux/1 -> deg2rad/1
  deg2rad/1 -> Fcn/1, Fcn1/1
  Fcn/1 -> Zero-Order Hold/1
  Fcn1/1 -> Zero-Order Hold1/1
  Zero-Order Hold/1 -> ms22g/1
  Zero-Order Hold1/1 -> ms22g1/1
  ms22g/1 -> Sum/2
  Random Number/1 -> Sum/1
  Random Number1/1 -> Sum1/2
  ms22g1/1 -> Sum1/1
  Sum1/1 -> Quantizer1/1
  Sum/1 -> Quantizer/1
  Quantizer/1 -> ax [g]/1
  Quantizer1/1 -> az [g]/1

== system lab4_S6_7_8_estimation_control/Balancing Robot Hardware Setup/Motion Processing Unit (MPU)/Gyroscope ==
  dot_q [deg/s] : Inport
  Quantizer2 : Quantizer  QuantizationInterval=sens.mpu.gyro.LSB2degs
  Random Number2 : RandomNumber  Variance=sens.mpu.gyro.noisevar  SampleTime=Ts
  Selector : Selector  InputPortWidth=2  IndexOptions=Index vector (dialog)  Indices=2  OutputSizes=1
  Sum2 : Sum  Inputs=++|
  Zero-Order Hold2 : ZeroOrderHold  SampleTime=Ts
  wy [deg/s] : Outport
  wires:
  Sum2/1 -> Quantizer2/1
  Zero-Order Hold2/1 -> Sum2/2
  Random Number2/1 -> Sum2/1
  Quantizer2/1 -> wy [deg/s]/1
  dot_q [deg/s]/1 -> Selector/1
  Selector/1 -> Zero-Order Hold2/1
